simulink model "controller13_jumping"  (R2023a)
settings: Solver=FixedStepAuto  StartTime=0.0  StopTime=mdl.exe_time  RelTol=1e-3
values from neighbouring files (symbols this model uses):
  ctr2 = ctr    [s1_setup.m]    (also in step1_setup.m; step1_setup_v1.m)
  lut = gen_lut    [s1_setup.m]    (also in thrust2voltage_lut_20230809.mat = ; thrust2voltage_lut_20230829.mat = )
  mdl = make_model(mdl,rsim)    [s1_setup.m]    (also in setup_controller_with_functions.m = make_model(flight_time); step1_setup.m; step1_setup_v1.m = make_model(flight_time,rsim))
undefined symbols (not defined in the file or in its folder): Angle, Axis, DiscIntNeverNeededParam, rjsim, servo_config, Standard_Devices, UDP_Protocol, use_simulation
libraries: simulink x25, sldrtlib x9, robotcorelib x8, dspmathops x3, dspswit3 x2, shared6dofsys x2, dspfdesign x2, sharedtransform x1, sharedutil x1, matrix_library x1, shared6dof x1, simulink_extras x1
(part 1 of 3)
settings Model: SimulationMode=external  ExtModeTrigDuration=1000001  Creator=SMRL  LastModifiedBy=SMRL
settings HardwareCC: ProdBitPerLong=64  ProdHWDeviceType=Intel->x86-64 (Linux 64)
settings RTWCC: Description=Simulink Desktop Real-Time  SystemTargetFile=sldrt.tlc  TemplateMakefile=sldrt.tmf  RTWCompilerOptimization=on
settings CodeAppCC: MaxIdLength=95
settings SimulinkDesktopRealTimeCC: TargetLibSuffix=_sldrt.a  TargetPreCompLibLocation=C:\Program Files\MATLAB\R2023a\toolbox\sldrt\lib\win64

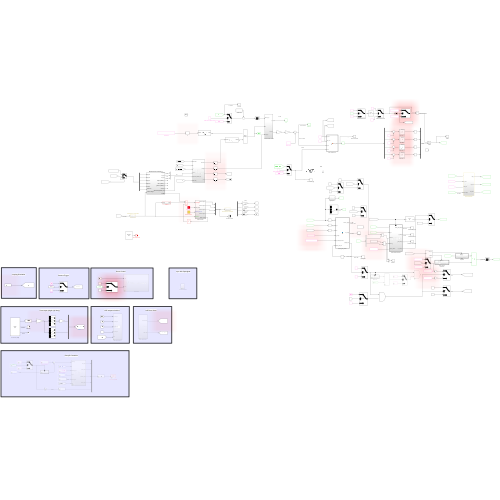
[thumbnail: Simulink's stored preview of the top-level diagram]
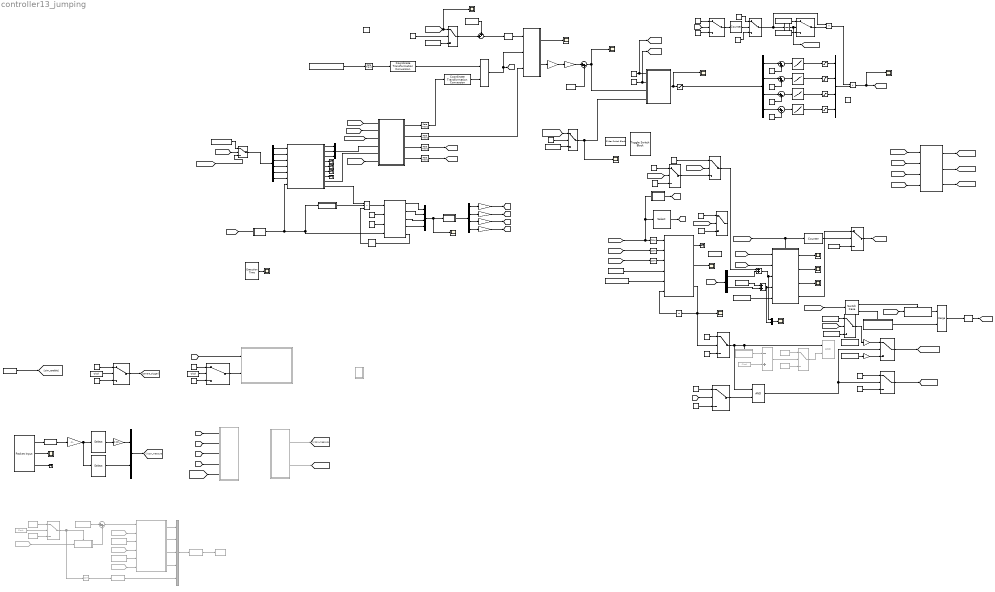
== system controller13_jumping ==
  note: Crazyflie Controller
  note: Jumping Simulation
  note: Vicon Input (single rigid body)
  note: Camera Trigger
  note: UDP output to Arduino
  note: correct
  note: correct
  note: Servo Control
  note: UDP from Vicon
  note: sync with Speedgoat
  AND1 : Logic  Commented=on  IconShape=distinctive  AllPortsSameDT=off  OutDataTypeStr=boolean
  AND2 : Logic  IconShape=distinctive  AllPortsSameDT=off  OutDataTypeStr=boolean
  Add{,2..5} (5 alike) : Sum  Inputs=|++
  Add1 : Sum
  Add6 : Sum  Commented=on  Inputs=-+
  Add7 : Sum  Inputs=++|
  Add8 : Sum  Commented=on  Inputs=|++
  Add9 : Sum
  Constant : Constant  Value=use_simulation
  Constant{1,17,34,36} (4 alike) : Constant
  Constant10 : Constant  Value=false
  Constant11 : Constant  Value=true
  Constant12 : Constant  Value=0.45
  Constant{2,13..16,18,35,37,42} (9 alike) : Constant  Value=0
  Constant19 : Constant  Value=mdl.leg_length
  Constant20 : Constant  Value=mdl.foot_altitude_threshold
  Constant21 : Constant  Value=true
  Constant22 : Constant  Value=false
  Constant23 : Constant  Value=true
  Constant24 : Constant  Value=false
  Constant25 : Constant  Commented=on  Value=false
  Constant26 : Constant  Commented=on  Value=true
  Constant27 : Constant  Value=mdl.high_thrust
  Constant28 : Constant  Value=mdl.low_thrust
  Constant29 : Constant  Value=mdl.desired_y
  Constant3 : Constant  Value=mdl.jumping_altitude
  Constant30 : Constant  Value=[0;0;1]
  Constant31 : Constant  Value=-0.01
  Constant32 : Constant  Commented=on  Value=0  OutDataTypeStr=double
  Constant33 : Constant  Commented=on  Value=true
  Constant38 : Constant  Value=[1600; 1600; 1600; 1600;]
  Constant39 : Constant  Commented=on  Value=false
  Constant4 : Constant  Value=mdl.desired_x
  Constant41 : Constant  Value=0.115
  Constant43 : Constant  Value=0.425
  Constant44 : Constant  Value=mdl.high_thrust
  Constant45 : Constant  Value=mdl.high_thrust2
  Constant46 : Constant  Value=ones(6,1)
  Constant5 : Constant  Value=200/4
  Constant6 : Constant  Value=0.025
  Constant7 : Constant  Value=0.043
  Constant8 : Constant  Value=[0;0;1]
  Constant9 : Constant  Value="[0.9995    0.0008   -0.0330; 0.0008    0.9989    0.0468; 0.0330   -0.0468    0.9984]"  VectorParams1D=off
  Coordinate Transformation Conversion : robotcorelib/Coordinate Transformation Conversion  InputRepresentation=Euler Angles  InputEulerSequence=XYZ  ShowTrVecInputPort=on  OutputRepresentation=Rotation Matrix  OutputEulerSequence=ZYX  ShowTrVecOutputPort=on  SimulateUsing=Interpreted execution
  Coordinate Transformation Conversion1 : robotcorelib/Coordinate Transformation Conversion  InputRepresentation=Euler Angles  InputEulerSequence=ZYX  ShowTrVecInputPort=on  OutputRepresentation=Rotation Matrix  OutputEulerSequence=ZYX  ShowTrVecOutputPort=on  SimulateUsing=Interpreted execution
  Counter1 : dspswit3/Counter  Direction=Up  CountEvent=Rising edge  CounterSize=8 bits  MaxCount=255  InitialCount=0  Output=Count  HitValue=32  ResetInput=off  SamplesPerFrame=1  Ts=1  CntDtype=double  HitDtype=Logical
  Counter2 : dspswit3/Counter  Direction=Up  CountEvent=Rising edge  CounterSize=8 bits  MaxCount=255  InitialCount=0  Output=Count  HitValue=32  ResetInput=off  SamplesPerFrame=1  Ts=1  CntDtype=double  HitDtype=Logical
  Data Type Conversion : DataTypeConversion  OutDataTypeStr=double  SaturateOnIntegerOverflow=off  RndMeth=Floor
  Data Type Conversion2 : DataTypeConversion  Commented=on  OutDataTypeStr=double  SaturateOnIntegerOverflow=off  RndMeth=Floor
  Data Type Conversion5 : DataTypeConversion  Commented=on  OutDataTypeStr=single  SaturateOnIntegerOverflow=off  RndMeth=Floor
  Delay3 : Delay  InitialCondition=1
  Demux1 : Demux  Outputs=6
  Demux2 : Demux
  Demux3 : Demux  Outputs=2
  Demux4 : Demux
  Digital Clock : DigitalClock  SampleTime=1/10000
  Digital Clock1 : DigitalClock  Commented=on  SampleTime=mdl.T
  Digital Clock3 : DigitalClock  SampleTime=1/2000
  Digital Clock5 : DigitalClock  Commented=on  SampleTime=1/100
  Discrete-Time Integrator : DiscreteIntegrator  SampleTime=-1  ICPrevOutput=DiscIntNeverNeededParam  ICPrevScaledInput=DiscIntNeverNeededParam
  Execution Time : sldrtlib/Target Profiling/Execution Time  ShowTaskTimes=off
  Flapping Freq(hz)1 : Constant  Value=ctr2.freq_vec  SampleTime=-1
  From15 : From  Commented=on  GotoTag=p_cf
  From3 : From  Commented=on  GotoTag=p_cf
  From4 : From  Commented=on  GotoTag=p_dot_cf
  From8 : From  Commented=on  GotoTag=yaw_cf
  Gain : Gain  Gain=1*10e-4
  Gain1 : Gain  Gain=28.5
  Gain2 : Gain  Gain=1/4
  Gain4 : Gain  Gain=1/4
  Gain7 : Gain  Gain=1/mdl.vicon.gain
  Gain8 : Gain  Gain=0.001
  Jumping Simulation : Subsystem
  Matrix Multiply : Product  Multiplication=Matrix(*)
  Measurement manager 2 : Subsystem  SystemSampleTime=mdl.T
  Merge : Merge  InitialOutput=[0; 0; 1]
  Mux : Mux  Inputs=2
  Mux1 : Mux  Inputs=2
  Mux3 : Mux  Commented=on  Inputs=5
  Mux4 : Mux
  Mux7 : Mux
  Mux9 : Mux  Inputs=3
  NOT : Logic  Commented=on  Operator=NOT  IconShape=distinctive  AllPortsSameDT=off  OutDataTypeStr=boolean
  Nemo Bee 10 : Lookup_n-D  NumberOfTableDimensions=1  BreakpointsForDimension1=lut.T4  Table=lut.v4  InternalRulePriority=Speed  RndMeth=Simplest
  Nemo Bee 12 : Lookup_n-D  NumberOfTableDimensions=1  BreakpointsForDimension1=lut.T1  Table=lut.v1  InternalRulePriority=Speed  RndMeth=Simplest
  Nemo Bee 14 : Lookup_n-D  NumberOfTableDimensions=1  BreakpointsForDimension1=lut.T3  Table=lut.v3  InternalRulePriority=Speed  RndMeth=Simplest
  Nemo Bee 6 : Lookup_n-D  NumberOfTableDimensions=1  BreakpointsForDimension1=lut.T2  Table=lut.v2  InternalRulePriority=Speed  RndMeth=Simplest
  Normalization1 : dspmathops/Normalization  NormType=Squared 2-norm  Bias=1e-10  NormOver=Each column  Dimension=1  roundingMode=Floor  overflowMode=off  accumDataTypeStr=Inherit: Same as product output  accumLastDataTypeStr=Inherit: Same as product output  outputDataTypeStr=Inherit: Same as product output  outputMin=[]  outputMax=[]  outputLastDataTypeStr=Inherit: Same as product output
  Normalization2 : dspmathops/Normalization  NormType=Squared 2-norm  Bias=1e-10  NormOver=Each column  Dimension=1  roundingMode=Floor  overflowMode=off  accumDataTypeStr=Inherit: Same as product output  accumLastDataTypeStr=Inherit: Same as product output  outputDataTypeStr=Inherit: Same as product output  outputMin=[]  outputMax=[]  outputLastDataTypeStr=Inherit: Same as product output
  Packet Input : sldrtlib/Packet Input  SampleTime=1/2000  MaxMissedTicks=100  ShowMissedTicks=off  YieldWhenWaiting=off  DrvName=Standard_Devices/UDP_Protocol  DrvAddress=18000  DrvOptions=[0 18385 49 57 50 46 49 54 56 46 49 54 56 46 49 52 54 0 0 0 0 0 0 0 0 0 0 0 0 0 0 0 0 0 0 0 0 0 0 0 0 0 0 0 0 0 0 0 0 0 0 0 0 0 0 0 0 0 0 0 0 0 0 0 0 0 0 0 0 0 0 0 0 0 0 0 0 0 0 0 0 0 0 0 0 0 0 0 0 0 0 0 0 0 0 0 0 0 0 0 0 0 0 0 0 0 0 0 0 0 0 0 0 0 0 0 0 0 0 0 0 0 0 0 0 0 0 0 0 0 0 0 0 0 0 0 0 0 0 0 0 0 0 0 0 0 0 0 0 0 0 0 0 0 0 0 0 0 0 0 0 0 0 0 0 0 0 0 0 0 0 0 0 0 0 0 0 0 0 0 0 0 0 0 0 0 0 0 0 0 0 0 0 0 0 0 0 0 0 0 0 0 0 0 0 0 0 0 0 0 0 0 0 0 0 0 0 0 0 0 0 0 0 0 0 0 0 0 0 0 0 0 0 0 0 0 0 0 0 0 0 0 0 0 0 0 0 0 0 0 0 0 0 0 0 0]  PacketSize=24  DataTypes='6*int32'  ShowReady=on  ShowError=on  PacketID=1  ByteOrder=2  ShowTimestamp=off
      settings: AttributesFormatString=UDP Protocol [18000]
  Packet Output1 : sldrtlib/Packet Output  Commented=on  SampleTime=1/100  MaxMissedTicks=100  ShowMissedTicks=off  YieldWhenWaiting=off  DrvName=Standard_Devices/UDP_Protocol  DrvAddress=24050  DrvOptions=[0 25010 49 54 57 46 50 53 52 46 49 54 50 46 49 54 56 0 0 0 0 0 0 0 0 0 0 0 0 0 0 0 0 0 0 0 0 0 0 0 0 0 0 0 0 0 0 0 0 0 0 0 0 0 0 0 0 0 0 0 0 0 0 0 0 0 0 0 0 0 0 0 0 0 0 0 0 0 0 0 0 0 0 0 0 0 0 0 0 0 0 0 0 0 0 0 0 0 0 0 0 0 0 0 0 0 0 0 0 0 0 0 0 0 0 0 0 0 0 0 0 0 0 0 0 0 0 0 0 0 0 0 0 0 0 0 0 0 0 0 0 0 0 0 0 0 0 0 0 0 0 0 0 0 0 0 0 0 0 0 0 0 0 0 0 0 0 0 0 0 0 0 0 0 0 0 0 0 0 0 0 0 0 0 0 0 0 0 0 0 0 0 0 0 0 0 0 0 0 0 0 0 0 0 0 0 0 0 0 0 0 0 0 0 0 0 0 0 0 0 0 0 0 0 0 0 0 0 0 0 0 0 0 0 0 0 0 0 0 0 0 0 0 0 0 0 0 0 0 0 0 0 0 0 0 0]  PacketSize=20  DataTypes='5*single'  ShowReady=off  ShowError=off  PacketID=1  ByteOrder=1  InitialValue=[]  FinalValue=[]
      settings: AttributesFormatString=UDP Protocol [24050]
  Product : Product
  RT{1,4..7} (5 alike) : RateTransition  Integrity=off  OutPortSampleTime=mdl.T
  Saturation : Saturate  UpperLimit=600  LowerLimit=0
  Saturation1 : Saturate  UpperLimit=1750  LowerLimit=0
  Saturation2 : Saturate  UpperLimit=1800  LowerLimit=0
  Saturation3 : Saturate  UpperLimit=1800  LowerLimit=0
  Saturation4 : Saturate  UpperLimit=1800  LowerLimit=0
  Selector2 : Selector  InputPortWidth=6  IndexOptions=Index vector (dialog)  Indices=[1:3]  OutputSizes=1
  Selector3 : Selector  InputPortWidth=6  IndexOptions=Index vector (dialog)  Indices=[4:6]  OutputSizes=1
  Selector4 : Selector  InputPortWidth=3  IndexOptions=Index vector (dialog)  Indices=[3]  OutputSizes=1
  Slider Switch : SliderSwitchBlock
      settings: Values={{'Off', 'On'}, [0 1]}
  Subsystem2 : Subsystem  Commented=on
  Subsystem3 : Subsystem  Commented=on
  Subsystem6 : Subsystem
  Switch : Switch  Criteria=u2 > Threshold  Threshold=2  SaturateOnIntegerOverflow=off  InputSameDT=off
  Switch Case : SwitchCase
  Switch{1..2,12,16} (4 alike) : Switch  Criteria=u2 > Threshold  SaturateOnIntegerOverflow=off  InputSameDT=off
  Switch10 : Switch  Commented=on  Threshold=mdl.powered_climbing_time  SaturateOnIntegerOverflow=off  InputSameDT=off
  Switch11 : Switch  Criteria=u2 ~= 0  Threshold=mdl.powered_climbing_time  SaturateOnIntegerOverflow=off  InputSameDT=off
  Switch13 : Switch  Criteria=u2 > Threshold  Threshold=4  SaturateOnIntegerOverflow=off  InputSameDT=off
  Switch14 : Switch  Commented=on  Criteria=u2 > Threshold  Threshold=1  SaturateOnIntegerOverflow=off  InputSameDT=off
  Switch15 : Switch  Criteria=u2 > Threshold  Threshold=3  SaturateOnIntegerOverflow=off  InputSameDT=off
  Switch3 : Switch  Criteria=u2 ~= 0  Threshold=mdl.powered_climbing_time  SaturateOnIntegerOverflow=off  InputSameDT=off
  Switch4 : Switch  Threshold=0.135  SaturateOnIntegerOverflow=off  InputSameDT=off
  Switch5 : Switch  Criteria=u2 > Threshold  Threshold=3  SaturateOnIntegerOverflow=off  InputSameDT=off
  Switch6 : Switch  Criteria=u2 > Threshold  Threshold=2  SaturateOnIntegerOverflow=off  InputSameDT=off
  Switch7 : Switch  Criteria=u2 > Threshold  Threshold=mdl.servo_drop_time  SaturateOnIntegerOverflow=off  InputSameDT=off
  Switch8 : Switch  Threshold=3  SaturateOnIntegerOverflow=off  InputSameDT=off
  Switch9 : Switch  Criteria=u2 > Threshold  Threshold=mdl.flight_time  SaturateOnIntegerOverflow=off  InputSameDT=off
  Terminator{,5,10..13} (6 alike) : Terminator
  Toggle Switch : ToggleSwitchBlock
      settings: Values={{'Off', 'On'}, [0 1]}
  Trigger time : Subsystem  Commented=on  TreatAsAtomicUnit=on
  UDP send to Arduino : Subsystem  Commented=on
  Unit Delay : UnitDelay  InitialCondition=1  SampleTime=-1  HasFrameUpgradeWarning=on
  Vicon UDP receive : Subsystem  Commented=on
  Zero-Order Hold4 : ZeroOrderHold  SampleTime=1/2000
  Zero-Order Hold5 : ZeroOrderHold  SampleTime=1/2000
  Zero-Order Hold6 : ZeroOrderHold  SampleTime=1/2000
  attitude bias2 : Constant  Value="[0.0008   -0.060   -0.045]"
  attitude bias3 : Constant  Value=[0;0;0]
  base_torque : Constant  Value=[0;0;0]
  c1 (JP1) : Gain  Gain=1.0033
  c2 (B1) : Gain  Gain=0.9899
  c3 (W1)1 : Gain  Gain=0.9850
  c4 (JP2) : Gain  Gain=0.9722
  constant1 : Constant  Value=0  OutDataTypeStr=boolean
  constant2 : Constant  OutDataTypeStr=boolean
  counter 2 : Subsystem
  data ready : Scope
  desired xy : Scope
  desired_position : Constant  Commented=on  Value=[0.0,0,0.3]
  desired_velocity : Constant  Commented=on  Value=[0,0,0]
  enable jumping attitude control : Constant
  enable jumping thrust control : Constant
  enable2 : Product  Inputs=**
  falling subsystem : Subsystem  TreatAsAtomicUnit=on
  foot height : Scope
  get xy ini : Subsystem
  height to enable control : Switch  Criteria=u2 > Threshold  Threshold=0.140  SaturateOnIntegerOverflow=off  InputSameDT=off
  height to enable control1 : Switch  Threshold=1  SaturateOnIntegerOverflow=off  InputSameDT=off
  high driving signal : Scope
  high execution time : Scope
  jumping state : Scope
  jumping_state_tracker : MATLAB Function  TreatAsAtomicUnit=on
  landing attitude controller : Subsystem
  motor thrusts (mgf) : Scope
  power_distribution_2 : MATLAB Function  TreatAsAtomicUnit=on
  predicted landing time : Scope
  predicted p landing : Scope
  predicted p_dot landing : Scope
  safety voltage : Constant  Value=max(ctr2.safety.volt)
  servo control : Subsystem  Commented=on
  signal generator1 : Subsystem  SystemSampleTime=mdl.T_high
  signal safety (no imag & NaN) : Subsystem
  stance climbing subsystem : Subsystem  TreatAsAtomicUnit=on
  sync with Speedgoat : Subsystem  Commented=on
  thrust control (mg) : Scope
  times1 : Product  Inputs=3  RndMeth=Zero
  torque_b : Scope
  voltage safety (no imag & NaN) : Subsystem
  voltages : Scope
  yaw-free attitude controller : Subsystem
  z_b : Scope
  z_b_desired : Scope
  wires:
  landing attitude controller/3(p_dot_landing) -> predicted p_dot landing/1  "p_dot_landing"
  jumping_state_tracker/2(foot_height) -> foot height/1  "foot_height"
  c3 (W1)1/1 -> [c3]
  yaw-free attitude controller/1(z_b) -> z_b/1  "z_b"
  c4 (JP2)/1 -> [c4]
  Nemo Bee 6/1 -> Saturation2/1
  Digital Clock1/1 -> Add6/2
  attitude bias3/1 -> Add7/1
  Constant34/1 -> height to enable control1/1
  Constant36/1 -> Switch7/1
  Switch7/1 -> servo control/2(enable)
  Switch8/1 -> AND2/1, Trigger time/Trigger, AND1/1
  times1/1 -> signal generator1/1(EnableSignal)
  safety voltage/1 -> signal generator1/2(safety voltage)
  Demux4/4 -> c4 (JP2)/1
  Coordinate Transformation Conversion/1 -> Matrix Multiply/2  "rotm"
  Measurement manager 2/9(enable) -> times1/1
  Counter1/1 -> height to enable control1/2
  Add2/1 -> Nemo Bee 12/1
  Merge/1 -> Normalization2/1  "z_b_desired"
  enable jumping attitude control/1 -> Switch12/2
  signal safety (no imag & NaN)/1(Output) -> Demux4/1
  Constant35/1 -> height to enable control1/3
  Measurement manager 2/3(Z (m)1) -> Mux9/3  "z (m)"
  Gain2/1 -> Switch11/1
  Switch/1 -> [camera_trigger]
  Add/1 -> power_distribution_2/3(torque), torque_b/1  "torque_b (mgf*m)"
  Constant37/1 -> Switch7/3
  Constant30/1 -> Switch12/3
  Demux4/3 -> c3 (W1)1/1
  [z_b] -> falling subsystem/1(In1)
  Trigger time/1(Out1) -> Add6/1
  Demux4/2 -> c2 (B1)/1
  Nemo Bee 12/1 -> Saturation1/1
  Switch9/1 -> Product/2
  Saturation/1 -> Demux2/1
  Add4/1 -> Nemo Bee 14/1
  height to enable control/1 -> Counter1/1
  Discrete-Time Integrator/1 -> [jumping_time], Switch9/2
  Switch12/1 -> Add7/2
  Add7/1 -> Normalization1/1
  [xy_ini] -> Demux3/1
  counter 2/1(enable) -> times1/2
  voltage safety (no imag & NaN)/1(Output) -> counter 2/1(voltage), signal generator1/4(Amplitude), Measurement manager 2/7(control voltage)
  Switch Case/1 -> falling subsystem/Action
  Normalization2/1 -> [z_b_desired]
  falling subsystem/1(Out1) -> Merge/1
  Digital Clock3/1 -> Switch7/2
  jumping_state_tracker/3(jumping_state) -> Switch8/2, jumping state/1, Unit Delay/1  "jumping_state"
  Constant3/1 -> landing attitude controller/5(jumping_altitude)
  Switch Case/2 -> stance climbing subsystem/Action
  Demux1/4 -> Measurement manager 2/4(alpha in)
  Constant5/1 -> Switch2/3
  Measurement manager 2/2(Y (m)1) -> Mux9/2  "y (m)"
  Constant28/1 -> Gain4/1
  [p] -> landing attitude controller/1(p)
  Normalization1/1 -> yaw-free attitude controller/1(desired_z_b)
  Saturation1/1 -> Mux4/1
  Gain4/1 -> Switch11/3
  Switch10/1 -> AND1/2
  Constant26/1 -> Switch10/3
  Saturation3/1 -> Mux4/3
  enable2/1 -> voltages/1, [voltages]  "voltages"
  Constant15/1 -> Add4/2
  Constant24/1 -> Switch8/3
  Constant23/1 -> Switch8/1
  Switch2/1 -> thrust control (mg)/1, power_distribution_2/4(thrust)  "thrust control (mg)"
  Constant25/1 -> Switch10/1
  [p_dot] -> Zero-Order Hold5/1
  Demux2/2 -> Add3/1
  power_distribution_2/1(motors_thrust) -> motor thrusts (mgf)/1, Saturation/1  "motor thrusts (mg)"
  stance climbing subsystem/1(Out1) -> Merge/2
  Constant19/1 -> jumping_state_tracker/4(leg_length)
  Demux4/1 -> c1 (JP1)/1
  [z] -> height to enable control/2
  Add6/1 -> Switch10/2
  Nemo Bee 14/1 -> Saturation3/1
  [p] -> get xy ini/1(In1), Selector4/1, Zero-Order Hold6/1
  enable jumping thrust control/1 -> Switch2/2
  Constant21/1 -> Switch9/3
  Constant18/1 -> height to enable control/1
  Nemo Bee 10/1 -> Saturation4/1
  Constant20/1 -> jumping_state_tracker/5(foot_alitutde_threshold)
  Constant13/1 -> Add2/2
  Constant14/1 -> Add3/2
  Constant17/1 -> height to enable control/3
  Constant16/1 -> Add5/2
  Saturation2/1 -> Mux4/2
  Demux2/3 -> Add4/1
  constant2/1 -> Switch/3
  Saturation4/1 -> Mux4/4
  Demux1/3 -> Measurement manager 2/3(Z(m) in)
  Demux1/2 -> Measurement manager 2/2(Y(m) in)
  Constant6/1 -> [roll_arm], power_distribution_2/1(roll_arm)
  signal generator1/1(D2A DriveSignal 1) -> Mux7/1
  Constant22/1 -> Switch9/1
  Add5/1 -> Nemo Bee 10/1
  Measurement manager 2/1(X (m)1) -> Mux9/1  "x (m)"
  Unit Delay/1 -> jumping_state_tracker/6(jumping_state_old)
  [p] -> servo control/1(p_raw)  "p_raw"
  yaw-free attitude controller/2(torque_b) -> Gain/1
  Product/1 -> enable2/1  "jumping control enable"
  signal generator1/5(Enable overload) -> Delay3/1
  Add3/1 -> Nemo Bee 6/1
  Mux7/1 -> high driving signal/1, signal safety (no imag & NaN)/1(In1)  "rbt2 driving signal"
  Demux2/1 -> Add2/1
  c2 (B1)/1 -> [c2]
  [jumping_thrust] -> Switch2/1
  [rotm] -> Zero-Order Hold4/1
  Gain/1 -> Gain1/1
  [p_dot] -> landing attitude controller/2(p_dot)
  Constant7/1 -> [pitch_arm], power_distribution_2/2(pitch_arm)
  constant1/1 -> Switch/1
  Demux1/1 -> Measurement manager 2/1(X(m) in)
  c1 (JP1)/1 -> [c1]
  Digital Clock/1 -> Switch/2
  landing attitude controller/1(landing_time_stamp) -> predicted landing time/1  "landing_time"
  Demux1/6 -> Measurement manager 2/6(gamma in)
  signal generator1/2(D2A DriveSignal 2) -> Mux7/2
  signal generator1/3(D2A DriveSignal 3) -> Mux7/3
  [z_b_desired] -> z_b_desired/1, Switch12/1  "z_b_desired"
  Demux1/5 -> Measurement manager 2/5(beta in)
  [voltages] -> voltage safety (no imag & NaN)/1(In1)  "rbt2 voltage"
  Delay3/1 -> times1/3
  Flapping Freq(hz)1/1 -> signal generator1/3(frequency_vec (hz))
  Measurement manager 2/7(XYZ (m)) -> Terminator5/1
  landing attitude controller/2(p_landing) -> predicted p landing/1  "p_landing"
  signal generator1/4(D2A DriveSignal 4) -> Mux7/4
  Demux2/4 -> Add5/1
  base_torque/1 -> Add/2
  Packet Input/1 -> Data Type Conversion/1
  Packet Input/2 -> data ready/1  "data ready"
  Packet Input/3 -> Terminator11/1  "data error"
  Data Type Conversion/1 -> Gain7/1
  Gain7/1 -> Selector3/1, Selector2/1
  Selector2/1 -> Gain8/1
  Gain8/1 -> Mux/1
  Selector3/1 -> Mux/2
  Mux/1 -> [vicon_measure]
  Constant/1 -> [sim_enable]
  Selector4/1 -> [z]  "p_raw"
  landing attitude controller/4(z_b_landing) -> Switch1/1
  Counter2/1 -> Switch1/2
  Constant8/1 -> Switch1/3
  Switch1/1 -> [z_b]
  Switch11/1 -> [jumping_thrust]  "thrust"
  Zero-Order Hold4/1 -> jumping_state_tracker/3(rotm)  "sim_p"
  Zero-Order Hold5/1 -> jumping_state_tracker/2(p_dot)  "sim_p"
  Zero-Order Hold6/1 -> jumping_state_tracker/1(p)  "sim_p"
  attitude bias2/1 -> RT1/1
  From3/1 -> Subsystem3/2(p)
  Subsystem3/1(roll_output) -> Mux3/1
  From8/1 -> Subsystem3/6(yaw)
  Data Type Conversion5/1 -> Packet Output1/1
  desired_velocity/1 -> Subsystem3/3(desired_p_dot)
  Digital Clock5/1 -> Switch14/2
  From15/1 -> Subsystem2/1(In1)  "p_raw"
  Subsystem3/2(pitch_output) -> Mux3/2
  Subsystem3/3(yawrate_output) -> Mux3/3
  From4/1 -> Subsystem3/4(p_dot)
  Mux3/1 -> Data Type Conversion5/1
  Subsystem3/4(thrust_output) -> Mux3/4
  Constant33/1 -> Switch14/1
  Constant32/1 -> Subsystem3/5(desired_yaw)  "disable"
  Add8/1 -> Subsystem3/1(desired_p)
  Constant39/1 -> Switch14/3
  NOT/1 -> Data Type Conversion2/1  "disable"
  desired_position/1 -> Add8/1
  Subsystem2/1(Out1) -> Add8/2
  Switch14/1 -> NOT/1, Subsystem2/Trigger
  Data Type Conversion2/1 -> Mux3/5
  Execution Time/1 -> high execution time/1
  Mux4/1 -> enable2/2  "voltages"
  [invR] -> Jumping Simulation/1(In1)
  [roll_arm] -> Jumping Simulation/2(roll_arm)
  [pitch_arm] -> Jumping Simulation/3(pitch_arm)
  [voltages] -> Jumping Simulation/4(rbt2 voltage)  "rbt2 voltage"
  Jumping Simulation/1(sim_p) -> [sim_p]
  Jumping Simulation/2(sim_rotm) -> [invR]
  Jumping Simulation/3(sim_rotm1) -> [sim_Eul_XYZ]
  Demux3/1 -> Add1/2
  Gain1/1 -> Add/1
  Measurement manager 2/8(alphs,beta,gamma (rad)) -> Subsystem6/5(alphs,beta,gamma (rad))
  RT7/1 -> Coordinate Transformation Conversion/1
  Measurement manager 2/6(gamma (radians)1) -> Terminator10/1
  Measurement manager 2/5(beta (radians)1) -> Terminator12/1
  Measurement manager 2/4(alpha (radians)1) -> Terminator13/1
  [sim_Eul_XYZ] -> Subsystem6/3(In3)
  [sim_enable] -> Subsystem6/1(sim enable)
  Mux9/1 -> Subsystem6/4(p raw)  "p raw"
  Subsystem6/1(Euler XYZ) -> RT7/1
  Subsystem6/2(omega b) -> RT4/1
  [sim_p] -> Subsystem6/2(In1)
  get xy ini/1(Out1) -> [xy_ini]
  [data_ready] -> Subsystem6/6(data ready)
  RT4/1 -> yaw-free attitude controller/3(omega_b)
  RT5/1 -> [p]
  Subsystem6/3("p ") -> RT5/1
  RT6/1 -> [p_dot]
  Subsystem6/4(p dot) -> RT6/1
  Constant1/1 -> Switch3/3
  Constant2/1 -> Switch3/1
  Switch3/1 -> [landing_trigger]  "thrust"
  [landing_trigger] -> landing attitude controller/Trigger, Counter2/1
  jumping_state_tracker/1(controller_trigger) -> Terminator/1  "controller_trigger"
  Add1/1 -> landing attitude controller/3(desired_x), Mux1/1
  Constant29/1 -> Add9/1
  Demux3/2 -> Add9/2
  Add9/1 -> Mux1/2, landing attitude controller/4(desired_y)
  [landing_trigger] -> Switch Case/1
  Matrix Multiply/1 -> yaw-free attitude controller/2(R), [rotm]
  [z] -> Switch4/2
  Constant10/1 -> Switch4/1
  Constant11/1 -> Switch4/3
  Switch4/1 -> AND2/2
  AND2/1 -> Switch11/2, Switch3/2
  height to enable control1/1 -> Product/1, Discrete-Time Integrator/1
  [jumping_time] -> Switch5/2
  Constant31/1 -> Switch5/3
  Constant12/1 -> Switch5/1
  Coordinate Transformation Conversion1/1 -> Matrix Multiply/1  "rotm"
  RT1/1 -> Coordinate Transformation Conversion1/1
  Mux1/1 -> desired xy/1
  Constant42/1 -> Switch6/3
  Constant41/1 -> Switch6/1
  [jumping_time] -> Switch6/2
  Switch6/1 -> Switch13/3
  Constant43/1 -> Switch13/1
  [jumping_time] -> Switch13/2
  [jumping_time] -> Switch15/2
  Constant44/1 -> Switch15/3
  Constant45/1 -> Switch15/1
  Switch15/1 -> Gain2/1
  Switch13/1 -> Add1/1
  [sim_enable] -> Switch16/2
  [vicon_measure] -> Switch16/3
  Switch16/1 -> Demux1/1
  Constant46/1 -> Switch16/1
  Vicon UDP receive/1(vicon measure) -> [vicon_measure]
  Vicon UDP receive/2(data ready) -> [data_ready]
  [c1] -> UDP send to Arduino/1(high voltage 1)
  [c2] -> UDP send to Arduino/2(high voltage 2)
  [c3] -> UDP send to Arduino/3(high voltage 3)
  [c4] -> UDP send to Arduino/4(high voltage 4)
  [camera_trigger] -> UDP send to Arduino/5(DO2)

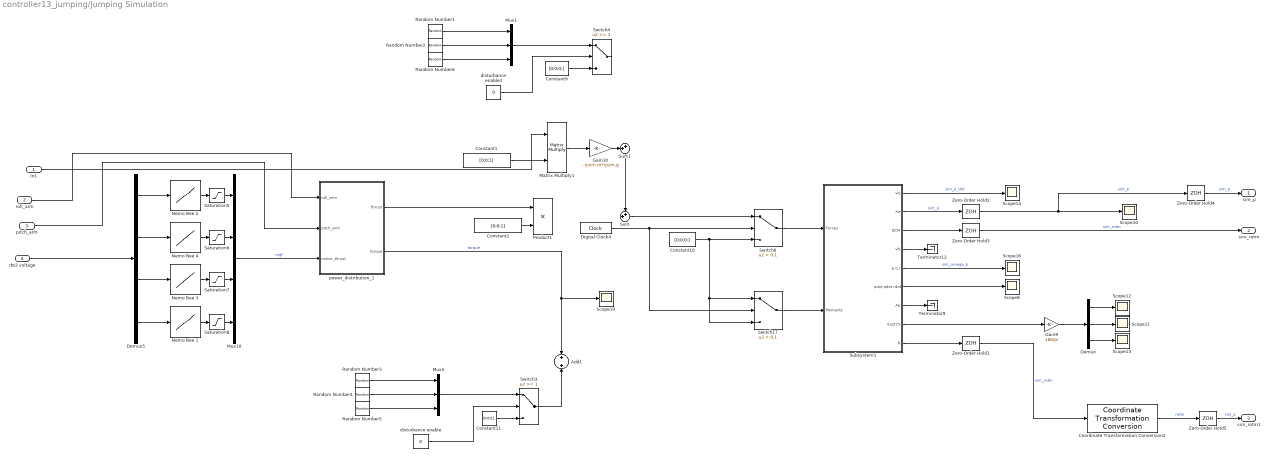
== system controller13_jumping/Jumping Simulation ==
  In1 : Inport
  roll_arm : Inport  Port=2
  pitch_arm : Inport  Port=3
  rbt2 voltage : Inport  Port=4
  Add1 : Sum
  Constant1 : Constant  Value=[0;0;1]
  Constant10 : Constant  Value=[0;0;0;]
  Constant11 : Constant  Value=[0;0;0;]
  Constant2 : Constant  Value=[0;0;1]
  Constant9 : Constant  Value=[0;0;0;]
  Coordinate Transformation Conversion2 : robotcorelib/Coordinate Transformation Conversion  InputRepresentation=Rotation Matrix  InputEulerSequence=XYZ  ShowTrVecInputPort=on  OutputRepresentation=Euler Angles  OutputEulerSequence=XYZ  ShowTrVecOutputPort=on  SimulateUsing=Interpreted execution
  Demux : Demux  Outputs=3
  Demux5 : Demux
  Digital Clock4 : DigitalClock  SampleTime=1/2000
  Gain10 : Gain  Gain=-rjsim.m*rjsim.g
  Gain9 : Gain  Gain=180/pi
  Matrix Multiply1 : Product  Multiplication=Matrix(*)
  Mux1 : Mux  Inputs=3
  Mux10 : Mux
  Mux5 : Mux  Inputs=3
  Nemo Bee 1 : Lookup_n-D  NumberOfTableDimensions=1  BreakpointsForDimension1=lut.v4  Table=lut.T4  InternalRulePriority=Speed  RndMeth=Simplest
  Nemo Bee 2 : Lookup_n-D  NumberOfTableDimensions=1  BreakpointsForDimension1=lut.v1  Table=lut.T1  InternalRulePriority=Speed  RndMeth=Simplest
  Nemo Bee 3 : Lookup_n-D  NumberOfTableDimensions=1  BreakpointsForDimension1=lut.v3  Table=lut.T3  InternalRulePriority=Speed  RndMeth=Simplest
  Nemo Bee 4 : Lookup_n-D  NumberOfTableDimensions=1  BreakpointsForDimension1=lut.v2  Table=lut.T2  InternalRulePriority=Speed  RndMeth=Simplest
  Product1 : Product
  Random Number1 : RandomNumber  Mean=rsim2.dist.x.mean  Variance=rsim2.dist.x.var  Seed=rsim2.dist.x.seed  SampleTime=1/2000
  Random Number2 : RandomNumber  Mean=rsim2.dist.y.mean  Variance=rsim2.dist.y.var  Seed=rsim2.dist.y.seed  SampleTime=1/2000
  Random Number3 : RandomNumber  Mean=rsim2.dist.wx.mean  Variance=rsim2.dist.wx.var  Seed=rsim2.dist.wx.seed  SampleTime=1/2000
  Random Number4 : RandomNumber  Mean=rsim2.dist.wy.mean  Variance=rsim2.dist.wy.var  Seed=rsim2.dist.wy.seed  SampleTime=1/2000
  Random Number5 : RandomNumber  Mean=rsim2.dist.wz.mean  Variance=rsim2.dist.wz.var  Seed=rsim2.dist.wz.seed  SampleTime=1/2000
  Random Number6 : RandomNumber  Mean=rsim2.dist.z.mean  Variance=rsim2.dist.z.var  Seed=rsim2.dist.z.seed  SampleTime=1/2000
  Saturation{5..8} (4 alike) : Saturate  UpperLimit=600  LowerLimit=0
  Scope{8,10..14,16,19} (8 alike) : Scope
  Subsystem1 : Subsystem
  Sum : Sum  Inputs=++|
  Sum1 : Sum  Inputs=++|
  Switch17 : Switch  Criteria=u2 > Threshold  Threshold=0.1  SaturateOnIntegerOverflow=off  InputSameDT=off
  Switch3 : Switch  Threshold=1  SaturateOnIntegerOverflow=off  InputSameDT=off
  Switch4 : Switch  Threshold=1  SaturateOnIntegerOverflow=off  InputSameDT=off
  Switch6 : Switch  Criteria=u2 > Threshold  Threshold=0.1  SaturateOnIntegerOverflow=off  InputSameDT=off
  Terminator12 : Terminator
  Terminator9 : Terminator
  Zero-Order Hold1 : ZeroOrderHold  SampleTime=1/2000
  Zero-Order Hold2 : ZeroOrderHold  SampleTime=1/2000
  Zero-Order Hold3 : ZeroOrderHold  SampleTime=1/2000
  Zero-Order Hold4 : ZeroOrderHold  SampleTime=1/400
  Zero-Order Hold5 : ZeroOrderHold  SampleTime=1/400
  disturbance enable : Constant  Value=0
  disturbance enable1 : Constant  Value=0
  power_distribution_1 : MATLAB Function  TreatAsAtomicUnit=on
  sim_p : Outport
  sim_rotm : Outport  Port=2
  sim_rotm1 : Outport  Port=3
  wires:
  Random Number5/1 -> Mux5/3
  Saturation6/1 -> Mux10/2
  disturbance enable/1 -> Switch3/2
  power_distribution_1/1(thrust) -> Product1/1
  Saturation8/1 -> Mux10/4
  Mux5/1 -> Switch3/1
  Digital Clock4/1 -> Switch17/2, Switch6/2
  Subsystem1/4(Vb) -> Terminator12/1
  Nemo Bee 1/1 -> Saturation8/1
  Subsystem1/2(Xe) -> Zero-Order Hold2/1  "sim_p"
  Constant11/1 -> Switch3/3
  Nemo Bee 4/1 -> Saturation6/1
  Constant2/1 -> Product1/2
  pitch_arm/1 -> power_distribution_1/2(pitch_arm)
  Gain9/1 -> Demux/1
  Constant1/1 -> Matrix Multiply1/2
  Demux5/3 -> Nemo Bee 3/1
  Subsystem1/7(Ab) -> Terminator9/1
  Random Number2/1 -> Mux1/2
  Mux10/1 -> power_distribution_1/3(motor_thrust)  "mgf"
  Random Number6/1 -> Mux1/3
  Subsystem1/6(pdot,qdot,rdot) -> Scope8/1
  Random Number3/1 -> Mux5/1
  Subsystem1/9(R) -> Zero-Order Hold1/1
  power_distribution_1/2(torque) -> Add1/1, Scope19/1  "torque"
  Gain10/1 -> Sum1/1
  Nemo Bee 3/1 -> Saturation7/1
  disturbance enable1/1 -> Switch4/2
  Zero-Order Hold2/1 -> Zero-Order Hold4/1, Scope10/1  "sim_p"
  Subsystem1/1(Ve) -> Scope14/1  "sim_p_dot"
  Demux/1 -> Scope12/1
  Demux5/1 -> Nemo Bee 2/1
  Matrix Multiply1/1 -> Gain10/1
  Switch6/1 -> Subsystem1/1(Forces)
  Random Number4/1 -> Mux5/2
  Saturation7/1 -> Mux10/3
  Switch3/1 -> Add1/2
  Demux/3 -> Scope13/1
  Demux5/2 -> Nemo Bee 4/1
  Switch17/1 -> Subsystem1/2(Moments)
  Mux1/1 -> Switch4/1
  Subsystem1/3(DCM) -> Zero-Order Hold3/1
  Constant9/1 -> Switch4/3
  In1/1 -> Matrix Multiply1/1
  Constant10/1 -> Switch17/1, Switch17/3, Switch6/3
  Sum1/1 -> Sum/1
  Demux5/4 -> Nemo Bee 1/1
  Subsystem1/5(p,q,r) -> Scope16/1  "sim_omega_b"
  Subsystem1/8(EulZYX) -> Gain9/1
  Saturation5/1 -> Mux10/1
  Sum/1 -> Switch6/1
  Random Number1/1 -> Mux1/1
  Demux/2 -> Scope11/1
  Nemo Bee 2/1 -> Saturation5/1
  roll_arm/1 -> power_distribution_1/1(roll_arm)
  Zero-Order Hold3/1 -> sim_rotm/1  "sim_rotm"
  Zero-Order Hold1/1 -> Coordinate Transformation Conversion2/1  "sim_rotm"
  rbt2 voltage/1 -> Demux5/1
  Coordinate Transformation Conversion2/1 -> Zero-Order Hold5/1  "rotm"
  Zero-Order Hold4/1 -> sim_p/1  "sim_p"
  Zero-Order Hold5/1 -> sim_rotm1/1  "sim_p"

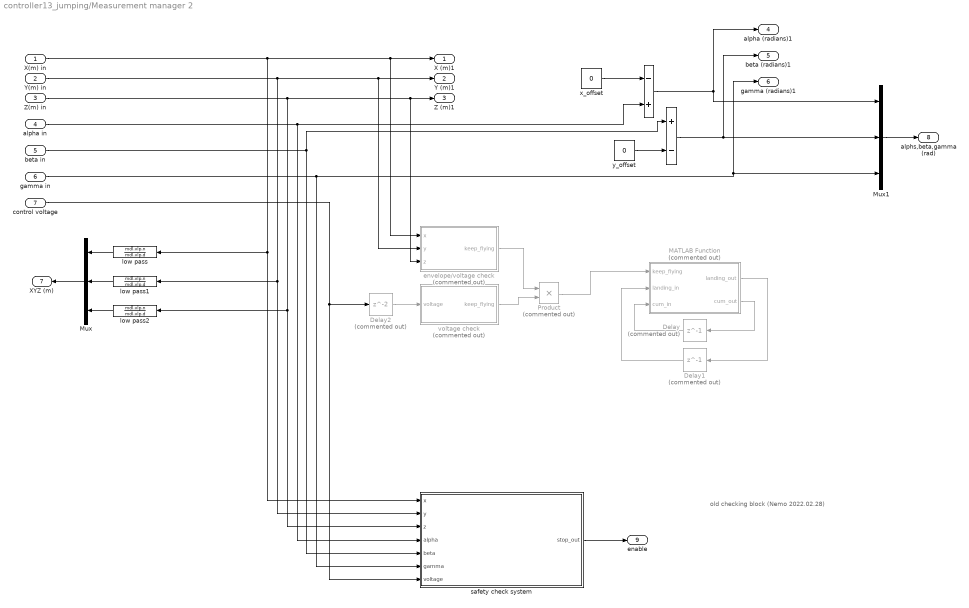
== system controller13_jumping/Measurement manager 2 ==
  note: old checking block (Nemo 2022.02.28)
  X(m) in : Inport
  Y(m) in : Inport  Port=2
  Z(m) in : Inport  Port=3
  alpha in : Inport  Port=4
  beta in : Inport  Port=5
  gamma in : Inport  Port=6
  control voltage : Inport  Port=7
  " " : Sum  Inputs=-+
  "  " : Sum  Inputs=+-
  Delay : Delay  Commented=on  DelayLength=1
  Delay1 : Delay  Commented=on  DelayLength=1
  Delay2 : Delay  Commented=on
  MATLAB Function : MATLAB Function  Commented=on  TreatAsAtomicUnit=on
  Mux : Mux  Inputs=3
  Mux1 : Mux  Inputs=3
  Product : Product  Commented=on
  envelope/voltage check : MATLAB Function  Commented=on  TreatAsAtomicUnit=on
  low pass : DiscreteTransferFcn  Numerator=mdl.vlp.n  Denominator=mdl.vlp.d
  low pass1 : DiscreteTransferFcn  Numerator=mdl.vlp.n  Denominator=mdl.vlp.d
  low pass2 : DiscreteTransferFcn  Numerator=mdl.vlp.n  Denominator=mdl.vlp.d
  safety check system : Subsystem
  voltage check : MATLAB Function  Commented=on  TreatAsAtomicUnit=on  SystemSampleTime=mdl.T
  x_offset : Constant  Value=0
  y_offset : Constant  Value=0
  X (m)1 : Outport
  Y (m)1 : Outport  Port=2
  Z (m)1 : Outport  Port=3
  alpha (radians)1 : Outport  Port=4
  beta (radians)1 : Outport  Port=5
  gamma (radians)1 : Outport  Port=6
  XYZ (m) : Outport  Port=7
  alphs,beta,gamma (rad) : Outport  Port=8
  enable : Outport  Port=9
  wires:
  X(m) in/1 -> safety check system/1(x), low pass/1, envelope/voltage check/1(x), X (m)1/1
  Y(m) in/1 -> safety check system/2(y), low pass1/1, envelope/voltage check/2(y), Y (m)1/1
  Z(m) in/1 -> safety check system/3(z), low pass2/1, envelope/voltage check/3(z), Z (m)1/1
  low pass1/1 -> Mux/2
  alpha in/1 -> safety check system/4(alpha), " "/2
  beta in/1 -> "  "/1, safety check system/5(beta)
  low pass/1 -> Mux/1
  low pass2/1 -> Mux/3
  Mux/1 -> XYZ (m)/1
  Mux1/1 -> alphs,beta,gamma (rad)/1
  y_offset/1 -> "  "/2
  x_offset/1 -> " "/1
  control voltage/1 -> Delay2/1, safety check system/7(voltage)
  safety check system/1(stop_out) -> enable/1
  " "/1 -> Mux1/1, alpha (radians)1/1
  "  "/1 -> beta (radians)1/1, Mux1/2
  gamma in/1 -> Mux1/3, gamma (radians)1/1, safety check system/6(gamma)
  Delay/1 -> MATLAB Function/3(cum_in)
  MATLAB Function/2(cum_out) -> Delay/1
  MATLAB Function/1(landing_out) -> Delay1/1
  Delay1/1 -> MATLAB Function/2(landing_in)
  envelope/voltage check/1(keep_flying) -> Product/1
  Delay2/1 -> voltage check/1(voltage)
  voltage check/1(keep_flying) -> Product/2
  Product/1 -> MATLAB Function/1(keep_flying)

== system controller13_jumping/Subsystem2 ==
  In1 : Inport
  Trigger : TriggerPort  VariantControl=Variant  PortDimensions=1
  Out1 : Outport
  wires:
  In1/1 -> Out1/1

== system controller13_jumping/Subsystem3 ==
  desired_p : Inport
  p : Inport  Port=2
  desired_p_dot : Inport  Port=3
  p_dot : Inport  Port=4
  desired_yaw : Inport  Port=5
  yaw : Inport  Port=6
  Add : Sum  Inputs=|+-
  Add1 : Sum  Inputs=|+-
  Add2 : Sum  Inputs=|++
  Add3 : Sum  Inputs=|++
  Add4 : Sum  Inputs=-+|
  Demux : Demux  Outputs=3
  Display : Display
  Gain : Gain
  MATLAB Function : MATLAB Function  TreatAsAtomicUnit=on
  Product : Product
  Product1 : Product
  d_gain : Constant  Value=[10, 10,25000]
  offset : Constant  Value=[0, 0,35000]
  p_gain : Constant  Value=[15, 15,20000]
  roll_output : Outport
  pitch_output : Outport  Port=2
  yawrate_output : Outport  Port=3
  thrust_output : Outport  Port=4
  wires:
  Product1/1 -> Add2/2
  p_gain/1 -> Product/2
  p/1 -> Add/2
  Demux/1 -> MATLAB Function/1(u_x)
  yaw/1 -> Add4/1, MATLAB Function/3(yaw)
  desired_p/1 -> Add/1
  Add/1 -> Product/1
  Add1/1 -> Product1/1
  p_dot/1 -> Add1/2
  Add2/1 -> Add3/1
  desired_p_dot/1 -> Add1/1
  d_gain/1 -> Product1/2
  offset/1 -> Add3/2
  Demux/2 -> MATLAB Function/2(u_y)
  Product/1 -> Add2/1
  Add3/1 -> Demux/1
  MATLAB Function/2(pitch) -> pitch_output/1  "pitch"
  Demux/3 -> Display/1, thrust_output/1  "thrust"
  MATLAB Function/1(roll) -> roll_output/1  "roll"
  Add4/1 -> Gain/1
  Gain/1 -> yawrate_output/1
  desired_yaw/1 -> Add4/2

== system controller13_jumping/Subsystem6 ==
  sim enable : Inport
  In1 : Inport  Port=2
  In3 : Inport  Port=3
  p raw : Inport  Port=4
  alphs,beta,gamma (rad) : Inport  Port=5
  data ready : Inport  Port=6
  Add1 : Sum  Inputs=+-
  Delay : Delay  DelayLength=25  InitialCondition=zeros(3,25)
  Digital Filter Design2 : dspfdesign/Digital Filter Design  mwdsp_browser_bugfix_var=off
  Eul_XYZ : Scope
  Gain : Gain  Gain=1/(25/10000)
  Subsystem4 : Subsystem
  Subsystem5 : Subsystem
  Switch1 : Switch  Criteria=u2 > Threshold  SaturateOnIntegerOverflow=off  InputSameDT=off
  Switch18 : Switch  Criteria=u2 > Threshold  SaturateOnIntegerOverflow=off  InputSameDT=off
  Switch5 : Switch  Criteria=u2 > Threshold  SaturateOnIntegerOverflow=off  InputSameDT=off
  Terminator8 : Terminator
  Terminator9 : Terminator
  omega_b : Scope
  p_dot : Scope
  p_raw : Scope
  Euler XYZ : Outport
  omega b : Outport  Port=2
  "p " : Outport  Port=3
  p dot : Outport  Port=4
  wires:
  Digital Filter Design2/1 -> omega b/1, omega_b/1  "omega b"
  ? -> ?  "omega_b"
  Switch5/1 -> Add1/1, Delay/1, Subsystem4/1(In1), "p "/1, p_raw/1  "p_raw"
  Switch18/1 -> Euler XYZ/1, Eul_XYZ/1, Subsystem5/1(euler_angles)  "Eul XYZ"
  Subsystem5/1(R) -> Terminator8/1
  sim enable/1 -> Subsystem5/3(sim enable), Switch1/2, Switch5/2, Switch18/2
  Subsystem5/3(Omega) -> Digital Filter Design2/1
  p raw/1 -> Switch5/3
  Subsystem5/2(Rdot) -> Terminator9/1
  alphs,beta,gamma (rad)/1 -> Switch18/3
  ? -> ?
  data ready/1 -> Subsystem5/2(data ready), Subsystem4/2(data ready)
  ? -> ?
  In1/1 -> Switch5/1
  In3/1 -> Switch18/1
  Delay/1 -> Add1/2
  Add1/1 -> Gain/1
  Gain/1 -> Switch1/1
  Subsystem4/1(p dot) -> Switch1/3
  Switch1/1 -> p dot/1, p_dot/1  "p_dot"

== system controller13_jumping/Trigger time ==
  Trigger : TriggerPort  VariantControl=(inherit)
  Digital Clock : DigitalClock  SampleTime=-1
  Out1 : Outport
  wires:
  Digital Clock/1 -> Out1/1

== system controller13_jumping/UDP send to Arduino ==
  high voltage 1 : Inport
  high voltage 2 : Inport  Port=2
  high voltage 3 : Inport  Port=3
  high voltage 4 : Inport  Port=4
  DO2 : Inport  Port=5
  HV amplifier gains : Subsystem
  Packet Output : sldrtlib/Packet Output  SampleTime=1/10000  MaxMissedTicks=100  ShowMissedTicks=off  YieldWhenWaiting=off  DrvName=Standard_Devices/UDP_Protocol  DrvAddress=22099  DrvOptions=[0 25000 49 54 57 46 50 53 52 46 49 48 51 46 52 50 0 0 0 0 0 0 0 0 0 0 0 0 0 0 0 0 0 0 0 0 0 0 0 0 0 0 0 0 0 0 0 0 0 0 0 0 0 0 0 0 0 0 0 0 0 0 0 0 0 0 0 0 0 0 0 0 0 0 0 0 0 0 0 0 0 0 0 0 0 0 0 0 0 0 0 0 0 0 0 0 0 0 0 0 0 0 0 0 0 0 0 0 0 0 0 0 0 0 0 0 0 0 0 0 0 0 0 0 0 0 0 0 0 0 0 0 0 0 0 0 0 0 0 0 0 0 0 0 0 0 0 0 0 0 0 0 0 0 0 0 0 0 0 0 0 0 0 0 0 0 0 0 0 0 0 0 0 0 0 0 0 0 0 0 0 0 0 0 0 0 0 0 0 0 0 0 0 0 0 0 0 0 0 0 0 0 0 0 0 0 0 0 0 0 0 0 0 0 0 0 0 0 0 0 0 0 0 0 0 0 0 0 0 0 0 0 0 0 0 0 0 0 0 0 0 0 0 0 0 0 0 0 0 0 0 0 0 0 0 0]  PacketSize=8  DataTypes='4*uint16'  ShowReady=off  ShowError=off  PacketID=1  ByteOrder=1  InitialValue=[]  FinalValue=[]
      settings: AttributesFormatString=UDP Protocol [22099]
  UDP send to Arduino DAC : Subsystem
  wires:
  UDP send to Arduino DAC/1(Output) -> Packet Output/1
  HV amplifier gains/2(DAC voltage 2) -> UDP send to Arduino DAC/2(DAC2)
  HV amplifier gains/4(DAC voltage 4) -> UDP send to Arduino DAC/4(DAC4)
  HV amplifier gains/1(DAC voltage 1) -> UDP send to Arduino DAC/1(DAC1)
  DO2/1 -> UDP send to Arduino DAC/5(DO2)
  HV amplifier gains/3(DAC voltage 3) -> UDP send to Arduino DAC/3(DAC3)
  high voltage 1/1 -> HV amplifier gains/1(high voltage 1)
  high voltage 3/1 -> HV amplifier gains/3(high voltage 3)
  high voltage 2/1 -> HV amplifier gains/2(high voltage 2)
  high voltage 4/1 -> HV amplifier gains/4(high voltage 4)

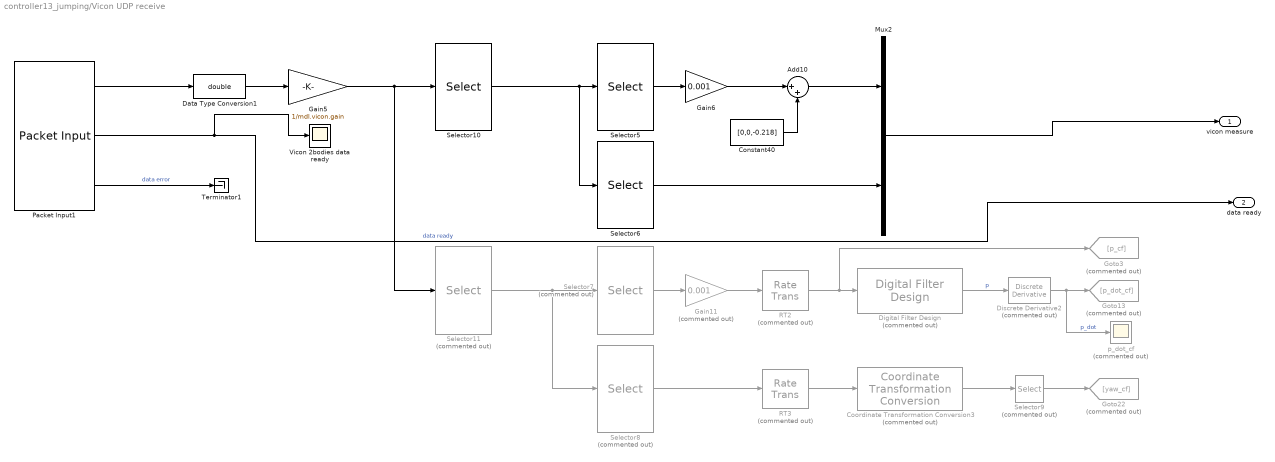
== system controller13_jumping/Vicon UDP receive ==
  Add10 : Sum  Inputs=|++
  Constant40 : Constant  Value=[0,0,-0.218]
  Coordinate Transformation Conversion3 : robotcorelib/Coordinate Transformation Conversion  Commented=on  InputRepresentation=Euler Angles  InputEulerSequence=XYZ  ShowTrVecInputPort=on  OutputRepresentation=Euler Angles  OutputEulerSequence=ZYX  ShowTrVecOutputPort=on  SimulateUsing=Interpreted execution
  Data Type Conversion1 : DataTypeConversion  OutDataTypeStr=double  SaturateOnIntegerOverflow=off  RndMeth=Floor
  Digital Filter Design : dspfdesign/Digital Filter Design  Commented=on  mwdsp_browser_bugfix_var=off
  Discrete Derivative2 : simulink/Discrete/Discrete Derivative  Commented=on  gainval=1.0  ICPrevScaledInput=0.0  OutMin=[]  OutMax=[]  OutDataType=fixdt(1, 16)  OutScaling=2^-10  DoSatur=off
  Gain11 : Gain  Commented=on  Gain=0.001
  Gain5 : Gain  Gain=1/mdl.vicon.gain
  Gain6 : Gain  Gain=0.001
  Goto13 : Goto  Commented=on  GotoTag=p_dot_cf
  Goto22 : Goto  Commented=on  GotoTag=yaw_cf
  Goto3 : Goto  Commented=on  GotoTag=p_cf
  Mux2 : Mux  Inputs=2
  Packet Input1 : sldrtlib/Packet Input  SampleTime=1/10000  MaxMissedTicks=100  ShowMissedTicks=off  YieldWhenWaiting=off  DrvName=Standard_Devices/UDP_Protocol  DrvAddress=18000  DrvOptions=[0 18885 49 54 57 46 50 53 52 46 49 54 56 46 49 52 54 0 0 0 0 0 0 0 0 0 0 0 0 0 0 0 0 0 0 0 0 0 0 0 0 0 0 0 0 0 0 0 0 0 0 0 0 0 0 0 0 0 0 0 0 0 0 0 0 0 0 0 0 0 0 0 0 0 0 0 0 0 0 0 0 0 0 0 0 0 0 0 0 0 0 0 0 0 0 0 0 0 0 0 0 0 0 0 0 0 0 0 0 0 0 0 0 0 0 0 0 0 0 0 0 0 0 0 0 0 0 0 0 0 0 0 0 0 0 0 0 0 0 0 0 0 0 0 0 0 0 0 0 0 0 0 0 0 0 0 0 0 0 0 0 0 0 0 0 0 0 0 0 0 0 0 0 0 0 0 0 0 0 0 0 0 0 0 0 0 0 0 0 0 0 0 0 0 0 0 0 0 0 0 0 0 0 0 0 0 0 0 0 0 0 0 0 0 0 0 0 0 0 0 0 0 0 0 0 0 0 0 0 0 0 0 0 0 0 0 0 0 0 0 0 0 0 0 0 0 0 0 0 0 0 0 0 0 0 0]  PacketSize=48  DataTypes='12*int32'  ShowReady=on  ShowError=on  PacketID=1  ByteOrder=2  ShowTimestamp=off
      settings: AttributesFormatString=UDP Protocol [18000]
  RT2 : RateTransition  Commented=on  Integrity=off  OutPortSampleTime=1/100
  RT3 : RateTransition  Commented=on  Integrity=off  OutPortSampleTime=1/100
  Selector10 : Selector  InputPortWidth=12  IndexOptions=Index vector (dialog)  Indices=[1:6]  OutputSizes=1
  Selector11 : Selector  Commented=on  InputPortWidth=12  IndexOptions=Index vector (dialog)  Indices=[7:12]  OutputSizes=1
  Selector5 : Selector  InputPortWidth=6  IndexOptions=Index vector (dialog)  Indices=[1:3]  OutputSizes=1
  Selector6 : Selector  InputPortWidth=6  IndexOptions=Index vector (dialog)  Indices=[4:6]  OutputSizes=1
  Selector7 : Selector  Commented=on  InputPortWidth=6  IndexOptions=Index vector (dialog)  Indices=[1:3]  OutputSizes=1
  Selector8 : Selector  Commented=on  InputPortWidth=6  IndexOptions=Index vector (dialog)  Indices=[4:6]  OutputSizes=1
  Selector9 : Selector  Commented=on  InputPortWidth=3  IndexOptions=Index vector (dialog)  Indices=[1]  OutputSizes=1
  Terminator1 : Terminator
  Vicon 2bodies data ready : Scope
  p_dot_cf : Scope  Commented=on
  vicon measure : Outport
  data ready : Outport  Port=2
  wires:
  Gain5/1 -> Selector11/1, Selector10/1
  Selector9/1 -> Goto22/1
  Discrete Derivative2/1 -> Goto13/1, p_dot_cf/1  "p_dot"
  Selector11/1 -> Selector8/1, Selector7/1
  RT3/1 -> Coordinate Transformation Conversion3/1
  Gain11/1 -> RT2/1
  Packet Input1/2 -> data ready/1, Vicon 2bodies data ready/1  "data ready"
  Digital Filter Design/1 -> Discrete Derivative2/1  "p"
  Selector6/1 -> Mux2/2
  Coordinate Transformation Conversion3/1 -> Selector9/1
  Selector5/1 -> Gain6/1
  Selector10/1 -> Selector6/1, Selector5/1
  Data Type Conversion1/1 -> Gain5/1
  Selector7/1 -> Gain11/1
  RT2/1 -> Goto3/1, Digital Filter Design/1
  Packet Input1/1 -> Data Type Conversion1/1
  Packet Input1/3 -> Terminator1/1  "data error"
  Selector8/1 -> RT3/1
  Add10/1 -> Mux2/1
  Constant40/1 -> Add10/2
  Gain6/1 -> Add10/1
  Mux2/1 -> vicon measure/1

== system controller13_jumping/counter 2 ==
  voltage : Inport
  Add : Sum  Commented=on  Inputs=+-
  Add1 : Sum  Commented=on
  Compare To Zero : simulink/Logic and Bit Operations/Compare To Zero  Commented=on  relop=<  OutDataTypeStr=uint8  ZeroCross=off
  Constant21 : Constant  Value=true
  Constant22 : Constant  Value=false
  Constant34 : Constant
  Constant35 : Constant  Value=0
  Delay : Delay  DelayLength=1  InitialCondition=[0;0;0;0;]
  Discrete-Time Integrator : DiscreteIntegrator  SampleTime=-1  ICPrevOutput=DiscIntNeverNeededParam  ICPrevScaledInput=DiscIntNeverNeededParam
  Discrete-Time Integrator1 : DiscreteIntegrator  SampleTime=-1  ICPrevOutput=DiscIntNeverNeededParam  ICPrevScaledInput=DiscIntNeverNeededParam
  Product : Product
  Product2 : Product  Commented=on  RndMeth=Zero
  Relational Operator : RelationalOperator  Commented=on  Operator=>  OutDataTypeStr=boolean  RndMeth=Simplest  InputSameDT=off
  Relational Operator1 : RelationalOperator  Operator=>  OutDataTypeStr=boolean  RndMeth=Simplest  InputSameDT=off
  SaturatingRamp : DiscreteIntegrator  Commented=on  gainval=1  SampleTime=-1  UpperSaturationLimit=1  LowerSaturationLimit=0  ICPrevOutput=DiscIntNeverNeededParam  ICPrevScaledInput=DiscIntNeverNeededParam
  Stop Simulation : Stop  Commented=on
  Sum of Elements : Sum  Inputs=+  OutDataTypeStr=double
  Switch9 : Switch  Criteria=u2 > Threshold  Threshold=mdl.flight_time-0.01  SaturateOnIntegerOverflow=off  InputSameDT=off
  constant : Constant  Commented=on
  height to enable control1 : Switch  Criteria=u2 > Threshold  SaturateOnIntegerOverflow=off  InputSameDT=off
  start delay compare : simulink/Logic and Bit Operations/Compare To Constant  Commented=on  relop=>  const=mdl.i_delay  OutDataTypeStr=uint8
  enable : Outport
  wires:
  SaturatingRamp/1 -> Relational Operator/1, Add/1, start delay compare/1
  Add/1 -> Compare To Zero/1
  start delay compare/1 -> Product2/1
  Compare To Zero/1 -> Product2/2
  constant/1 -> Add1/1, SaturatingRamp/1
  Relational Operator/1 -> Stop Simulation/1
  Add1/1 -> Relational Operator/2
  voltage/1 -> Delay/1, Relational Operator1/1
  Delay/1 -> Relational Operator1/2
  Constant34/1 -> height to enable control1/1
  Constant35/1 -> height to enable control1/3
  Sum of Elements/1 -> Discrete-Time Integrator1/1
  Constant22/1 -> Switch9/1
  Switch9/1 -> Product/2
  Constant21/1 -> Switch9/3
  height to enable control1/1 -> Product/1, Discrete-Time Integrator/1
  Discrete-Time Integrator/1 -> Switch9/2
  Relational Operator1/1 -> Sum of Elements/1
  Product/1 -> enable/1  "jumping control enable"
  Discrete-Time Integrator1/1 -> height to enable control1/2

== system controller13_jumping/falling subsystem ==
  In1 : Inport
  Action Port : ActionPort  ActionPortLabel=case [ 1 ]:
  Out1 : Outport
  wires:
  In1/1 -> Out1/1

== system controller13_jumping/get xy ini ==
  In1 : Inport
  Constant12 : Constant  Value=true
  Constant31 : Constant  Value=false
  Digital Clock2 : DigitalClock  SampleTime=1/2000
  IC : InitialCondition  Value=[0;0]
  Selector1 : Selector  InputPortWidth=3  IndexOptions=Index vector (dialog)  Indices=[1 2]  OutputSizes=1
  Subsystem : Subsystem
  Switch13 : Switch  Criteria=u2 > Threshold  Threshold=0.1  SaturateOnIntegerOverflow=off  InputSameDT=off
  Out1 : Outport
  wires:
  Switch13/1 -> Subsystem/Trigger
  Digital Clock2/1 -> Switch13/2
  In1/1 -> Subsystem/1(In1)
  Constant31/1 -> Switch13/3
  Subsystem/1(Out1) -> Selector1/1
  Selector1/1 -> IC/1  "p_raw"
  Constant12/1 -> Switch13/1
  IC/1 -> Out1/1

== system controller13_jumping/landing attitude controller ==
  p : Inport
  p_dot : Inport  Port=2
  desired_x : Inport  Port=3
  desired_y : Inport  Port=4
  jumping_altitude : Inport  Port=5
  Trigger : TriggerPort  VariantControl=(inherit)  PortDimensions=1
  Constant10 : Constant  Value=mdl.k2
  Constant11 : Constant  Value=mdl.g
  Constant12 : Constant  Value=mdl.leg_length
  Constant5 : Constant  Value=mdl.g
  Constant6 : Constant  Value=mdl.velocity_limit_ratio
  Digital Clock : DigitalClock  SampleTime=-1
  Gain1 : Gain  Gain=mdl.k3
  Sqrt : Sqrt
  Square : Math  Operator=square
  Sum of Elements : Sum  Inputs=+
  inverse_jumping_model : MATLAB Function  TreatAsAtomicUnit=on
  jumping_planning : MATLAB Function  TreatAsAtomicUnit=on
  landing_state_predictiction : MATLAB Function  TreatAsAtomicUnit=on
  landing_time_stamp : Outport
  p_landing : Outport  Port=2
  p_dot_landing : Outport  Port=3
  z_b_landing : Outport  Port=4
  wires:
  Sum of Elements/1 -> Sqrt/1
  p/1 -> landing_state_predictiction/2(p)
  landing_state_predictiction/3(landing_time_stamp) -> landing_time_stamp/1
  Digital Clock/1 -> landing_state_predictiction/1(time)
  Square/1 -> Sum of Elements/1
  inverse_jumping_model/1(landing_attitude_z_b) -> z_b_landing/1
  Constant10/1 -> inverse_jumping_model/3(k2)
  landing_state_predictiction/2(p_landing) -> p_landing/1, jumping_planning/4(p_landing)
  Gain1/1 -> jumping_planning/3(p_dot_TK)
  jumping_planning/1(takeoff_velocity) -> inverse_jumping_model/2(p_dot_takeoff)
  Constant5/1 -> jumping_planning/1(g)
  landing_state_predictiction/1(p_dot_landing) -> p_dot_landing/1, Square/1, inverse_jumping_model/1(p_dot_landing)
  Constant6/1 -> jumping_planning/2(velocity_limit_ratio)
  Constant12/1 -> landing_state_predictiction/5(leg_length)
  Constant11/1 -> landing_state_predictiction/4(g)
  p_dot/1 -> landing_state_predictiction/3(p_dot)
  Sqrt/1 -> Gain1/1
  desired_x/1 -> jumping_planning/5(desired_x)
  jumping_altitude/1 -> jumping_planning/7(jumping_altitude)
  desired_y/1 -> jumping_planning/6(desired_y)

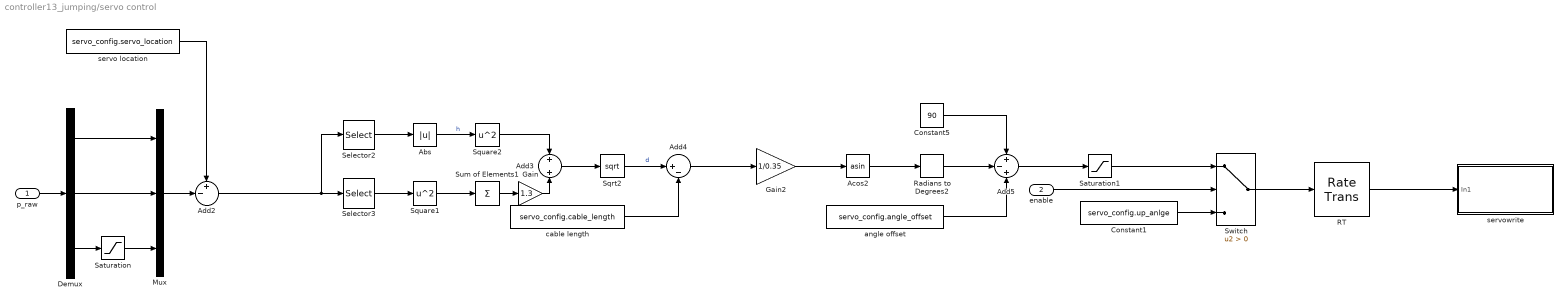
== system controller13_jumping/servo control ==
  p_raw : Inport
  enable : Inport  Port=2
  Abs : Abs  SaturateOnIntegerOverflow=off
  Acos2 : Trigonometry  Operator=asin  OutputSignalType=real
  Add2 : Sum  Inputs=+-|
  Add3 : Sum  Inputs=+|+
  Add4 : Sum  Inputs=|+-
  Add5 : Sum  Inputs=+-+
  Constant1 : Constant  Value=servo_config.up_anlge
  Constant5 : Constant  Value=90
  Demux : Demux  Outputs=3
  Gain : Gain  Gain=1.3
  Gain2 : Gain  Gain=1/0.35
  Mux : Mux  Inputs=3
  RT : RateTransition  Integrity=off  OutPortSampleTime=1/400
  Radians to Degrees2 : simulink_extras/Transformations/Radians to Degrees
  Saturation : Saturate  UpperLimit=0.8  LowerLimit=servo_config.z_lower_limit
  Saturation1 : Saturate  UpperLimit=90+45  LowerLimit=50
  Selector2 : Selector  InputPortWidth=3  IndexOptions=Index vector (dialog)  Indices=[3]  OutputSizes=1
  Selector3 : Selector  InputPortWidth=3  IndexOptions=Index vector (dialog)  Indices=[1 2]  OutputSizes=1
  Sqrt2 : Sqrt
  Square1 : Math  Operator=square
  Square2 : Math  Operator=square
  Sum of Elements1 : Sum  Inputs=+
  Switch : Switch  Criteria=u2 > Threshold  SaturateOnIntegerOverflow=off  InputSameDT=off
  angle offset : Constant  Value=servo_config.angle_offset
  cable length : Constant  Value=servo_config.cable_length
  servo location : Constant  Value=servo_config.servo_location
  servowrite : Subsystem
  wires:
  angle offset/1 -> Add5/3
  Add2/1 -> Selector3/1, Selector2/1
  Radians to Degrees2/1 -> Add5/2
  Sum of Elements1/1 -> Gain/1
  Sqrt2/1 -> Add4/1  "d"
  Add5/1 -> Saturation1/1
  servo location/1 -> Add2/1
  Square1/1 -> Sum of Elements1/1
  cable length/1 -> Add4/2
  Gain2/1 -> Acos2/1
  Abs/1 -> Square2/1  "h"
  Add4/1 -> Gain2/1
  Square2/1 -> Add3/1
  Acos2/1 -> Radians to Degrees2/1
  Selector3/1 -> Square1/1
  Constant5/1 -> Add5/1
  Add3/1 -> Sqrt2/1
  Saturation1/1 -> Switch/1
  Constant1/1 -> Switch/3
  Selector2/1 -> Abs/1
  Mux/1 -> Add2/2
  Demux/2 -> Mux/2
  Demux/1 -> Mux/1
  p_raw/1 -> Demux/1
  Demux/3 -> Saturation/1
  Saturation/1 -> Mux/3
  enable/1 -> Switch/2
  Switch/1 -> RT/1
  RT/1 -> servowrite/1(In1)
  Gain/1 -> Add3/2
